simulink model "SimulatorSpencer"  (R2024a)
settings: Solver=VariableStepAuto  StartTime=0.0  StopTime=inf  MaxStep=1  RelTol=1e-5
model workspace (MAT data in the model file):
  A = 10
values from neighbouring files (symbols this model uses):
  CheckBox = modes(i)    [ACSModeSequence.m]    (also in Constants_gui.m = LampModes(i))
  I = [3000 0 0 ... (first row only)    [Constants_gui.m]    (also in constants.m; mbi.m = [15, .25, .20; set_up_HW7.m = I-Id; setupConstantRateSDA.m)
  invI = inv(I)    [Constants_gui.m]    (also in constants.m; mbi.m; set_up_HW7.m; setupConstantRateSDA.m)
  q_init = q_init/norm(q_init)    [Constants_gui.m]    (also in constants.m = [-0.5 -0.5 -0.5 0.5]; mbi.m = [0 0 0 1]'; set_up_HW7.m = [0 0 0 1]'; setupConstantRateSDA.m)
  wbn_init = pi/30*[0 0 0]'    [Constants_gui.m]    (also in constants.m = pi/180 * [0.1; 0.2; 0.15]; mbi.m = [0 0 0]'; set_up_HW7.m = pi/30*[0 0 .01]'; setupConstantRateSDA.m)
  wn = 0.01    [Constants_gui.m]    (also in constants.m = 0.05; setupConstantRateSDA.m = 0.05)
  zet = .7071    (= 0.7071)    [Constants_gui.m]    (also in constants.m; setupConstantRateSDA.m)
libraries: aerolibutil x9, sharedutil x8, sharedtransform x2, sldrtlib x1, dspinverses x1, vrlib x1
(part 3 of 4)

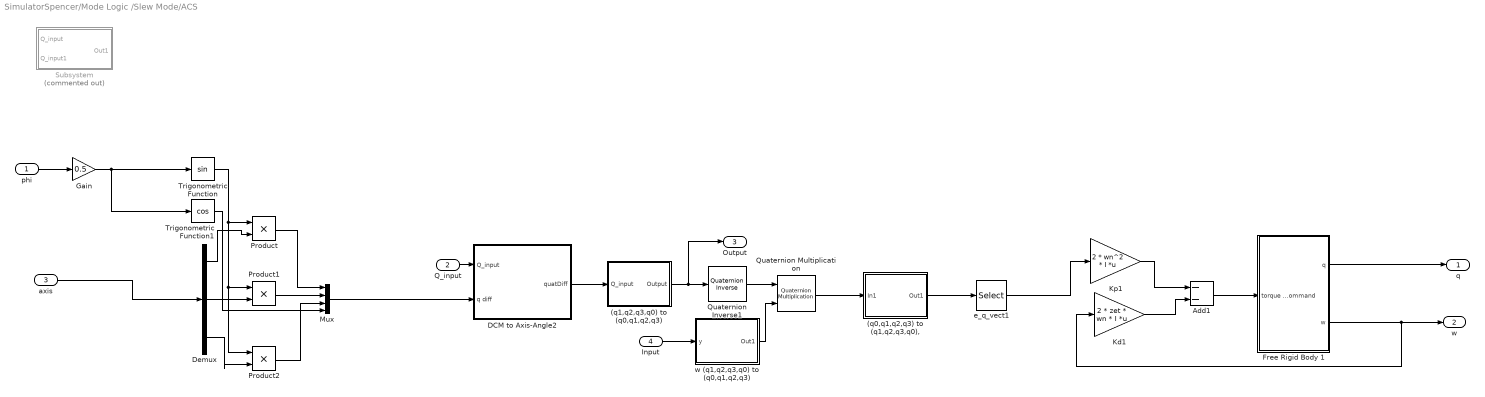
== system SimulatorSpencer/Mode Logic /Slew Mode/ACS ==
  phi : Inport
  Q_input : Inport  Port=2
  axis : Inport  Port=3
  Input : Inport  Port=4
  (q0,q1,q2,q3) to (q1,q2,q3,q0), : Subsystem
  "(q1,q2,q3,q0) to (q0,q1,q2,q3) " : Subsystem
  Add1 : Sum  Inputs=--
  DCM to Axis-Angle2 : Subsystem
  Demux : Demux  Outputs=3
  Free Rigid Body 1 : Subsystem
  Gain : Gain  Gain=0.5
  Kd1 : Gain  Gain=2 * zet * wn * I  Multiplication=Matrix(K*u)  SaturateOnIntegerOverflow=on  OutDataTypeStr=Inherit: Same as input  ParamDataTypeStr=Inherit: Same as input
  Kp1 : Gain  Gain=2 * wn^2 * I  Multiplication=Matrix(K*u)  SaturateOnIntegerOverflow=on  OutDataTypeStr=Inherit: Same as input  ParamDataTypeStr=Inherit: Same as input
  Mux : Mux
  Product : Product
  Product1 : Product
  Product2 : Product
  Quaternion Inverse1 : aerolibutil/Quaternion Inverse
  Quaternion Multiplication : aerolibutil/Quaternion Multiplication
  Subsystem : Subsystem  Commented=on
  Trigonometric Function : Trigonometry
  Trigonometric Function1 : Trigonometry  Operator=cos
  e_q_vect1 : Selector  InputPortWidth=4  IndexOptions=Index vector (dialog)  Indices=[1 2 3]  OutputSizes=1
  "w (q1,q2,q3,q0) to (q0,q1,q2,q3) " : Subsystem
      settings: PortSchema="{\"entries\":[{\"content\":{\"sides\":[{\"content\":{\"connectorIds\":[\"Out1\"]},\"type\":\"ConnectorPlacement.EquallySpacedRectSide\",\"uuid\":\"97b477ad-5663-4010-b344-d27b8ec095be\"},{\"content\":{\"connectorIds\":[\"In1\"],\"side\":\"RIGHT\"},\"type\":\"ConnectorPlacement.EquallySpacedRectSide\",\"uuid\":\"41fe4029-0263-4427-bdfc-3c26258b8a65\"},{\"content\":{\"side\":\"TOP\"},\"type\":\"ConnectorPlacement.EquallySpacedRectSide\",\"uuid\":\"9fb3a03d-539a-4245-bd7d-8174d3d0797f\"}]},\"type\":\"ConnectorPlacement.EquallySpacedConnector\",\"uuid\":\"44222554-f3ae-4bc6-b92c-7571a5ce84f7\"}],\"packageUris\":[\"http://schema.mathworks.com/mf0/Connector/R2020b\"],\"version\":\"1.0\"}"
  q : Outport
  w : Outport  Port=2
  Output : Outport  Port=3
  wires:
  Product1/1 -> Mux/2
  Product2/1 -> Mux/3
  Demux/1 -> Product/2
  Gain/1 -> Trigonometric Function1/1, Trigonometric Function/1
  Product/1 -> Mux/1
  phi/1 -> Gain/1
  Demux/2 -> Product1/2
  Demux/3 -> Product2/2
  Trigonometric Function1/1 -> Mux/4
  Trigonometric Function/1 -> Product2/1, Product1/1, Product/1
  axis/1 -> Demux/1
  Q_input/1 -> DCM to Axis-Angle2/1(Q_input)
  Mux/1 -> DCM to Axis-Angle2/2(q diff)
  Quaternion Multiplication/1 -> (q0,q1,q2,q3) to (q1,q2,q3,q0),/1(In1)
  "w (q1,q2,q3,q0) to (q0,q1,q2,q3) "/1(Out1) -> Quaternion Multiplication/2
  Quaternion Inverse1/1 -> Quaternion Multiplication/1
  Add1/1 -> Free Rigid Body 1/1(torque command)
  Kd1/1 -> Add1/2
  Free Rigid Body 1/2(w) -> w/1, Kd1/1
  "(q1,q2,q3,q0) to (q0,q1,q2,q3) "/1(Output) -> Output/1, Quaternion Inverse1/1
  e_q_vect1/1 -> Kp1/1
  DCM to Axis-Angle2/1(quatDiff) -> "(q1,q2,q3,q0) to (q0,q1,q2,q3) "/1(Q_input)
  (q0,q1,q2,q3) to (q1,q2,q3,q0),/1(Out1) -> e_q_vect1/1
  Kp1/1 -> Add1/1
  Free Rigid Body 1/1(q) -> q/1
  Input/1 -> "w (q1,q2,q3,q0) to (q0,q1,q2,q3) "/1(y)

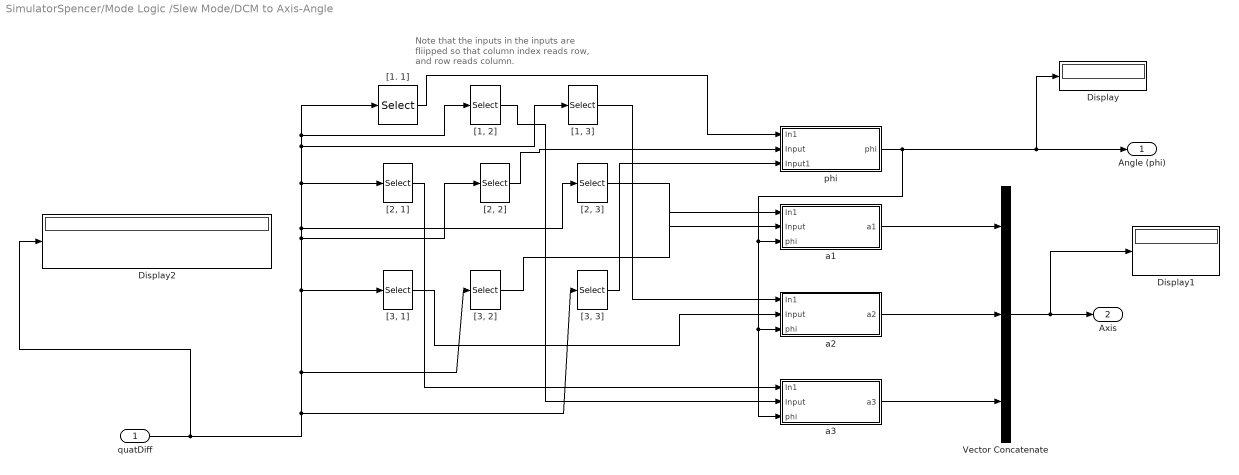
== system SimulatorSpencer/Mode Logic /Slew Mode/DCM to Axis-Angle ==
  note: Note that the inputs in the inputs are fliipped so that column index reads row, and row reads column.
  quatDiff : Inport
  Display : Display
  Display1 : Display
  Display2 : Display
  Vector Concatenate : Concatenate  NumInputs=3
  "[1, 2]" : Selector  NumberOfDimensions=2  InputPortWidth=3  IndexOptions=Index vector (dialog),Index vector (dialog)  Indices=2,1  OutputSizes=1,1
  "[1, 3]" : Selector  NumberOfDimensions=2  InputPortWidth=3  IndexOptions=Index vector (dialog),Index vector (dialog)  Indices=3,1  OutputSizes=1,1
  "[1. 1]" : Selector  NumberOfDimensions=2  InputPortWidth=3  IndexOptions=Index vector (dialog),Index vector (dialog)  Indices=1,1  OutputSizes=1,1
  "[2, 1]" : Selector  NumberOfDimensions=2  InputPortWidth=3  IndexOptions=Index vector (dialog),Index vector (dialog)  Indices=1,2  OutputSizes=1,1
  "[2, 2]" : Selector  NumberOfDimensions=2  InputPortWidth=3  IndexOptions=Index vector (dialog),Index vector (dialog)  Indices=2,2  OutputSizes=1,1
  "[2, 3]" : Selector  NumberOfDimensions=2  InputPortWidth=3  IndexOptions=Index vector (dialog),Index vector (dialog)  Indices=3,2  OutputSizes=1,1
  "[3, 1]" : Selector  NumberOfDimensions=2  InputPortWidth=3  IndexOptions=Index vector (dialog),Index vector (dialog)  Indices=1,3  OutputSizes=1,1
  "[3, 2]" : Selector  NumberOfDimensions=2  InputPortWidth=3  IndexOptions=Index vector (dialog),Index vector (dialog)  Indices=2,3  OutputSizes=1,1
  "[3, 3]" : Selector  NumberOfDimensions=2  InputPortWidth=3  IndexOptions=Index vector (dialog),Index vector (dialog)  Indices=3,3  OutputSizes=1,1
  a1 : Subsystem
  a2 : Subsystem
  a3 : Subsystem
  phi : Subsystem
  Angle (phi) : Outport
  Axis : Outport  Port=2
  wires:
  Vector Concatenate/1 -> Display1/1, Axis/1
  "[3, 3]"/1 -> phi/3(Input1)
  "[2, 3]"/1 -> a1/2(Input)
  "[1, 3]"/1 -> a2/1(In1)
  a2/1(a2) -> Vector Concatenate/2
  "[2, 2]"/1 -> phi/2(Input)
  "[1, 2]"/1 -> a3/2(Input)
  "[1. 1]"/1 -> phi/1(In1)
  "[2, 1]"/1 -> a3/1(In1)
  "[3, 1]"/1 -> a2/2(Input)
  "[3, 2]"/1 -> a1/1(In1)
  quatDiff/1 -> Display2/1, "[3, 2]"/1, "[3, 1]"/1, "[2, 1]"/1, "[1, 3]"/1, "[1, 2]"/1, "[1. 1]"/1, "[2, 3]"/1, "[2, 2]"/1, "[3, 3]"/1
  phi/1(phi) -> Angle (phi)/1, Display/1, a3/3(phi), a2/3(phi), a1/3(phi)
  a3/1(a3) -> Vector Concatenate/3
  a1/1(a1) -> Vector Concatenate/1

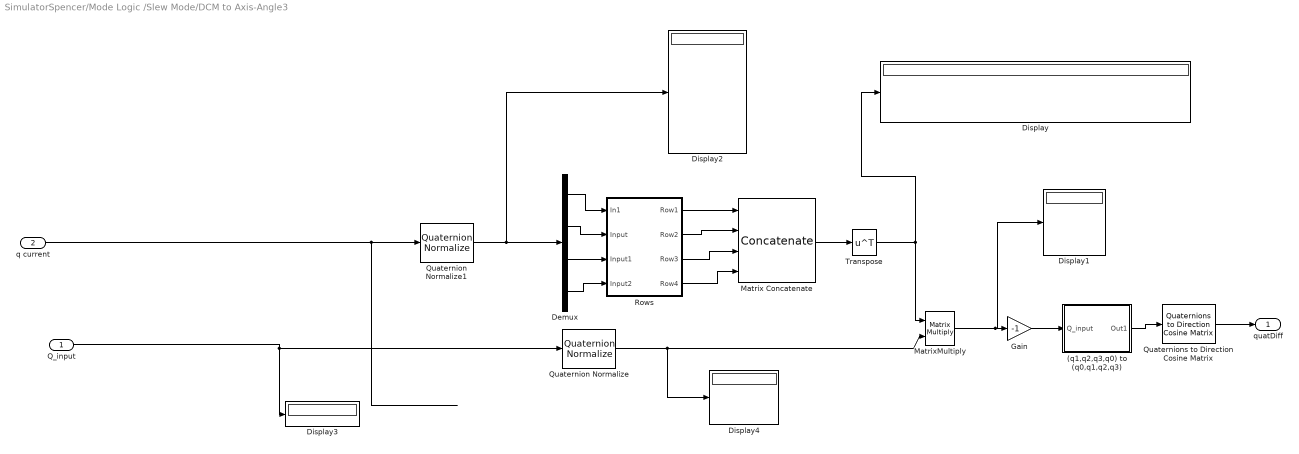
== system SimulatorSpencer/Mode Logic /Slew Mode/DCM to Axis-Angle3 ==
  Q_input : Inport
  q current : Inport  Port=2
  "(q1,q2,q3,q0) to (q0,q1,q2,q3) " : Subsystem
  Demux : Demux
  Display{,1..4} (5 alike) : Display
  Gain : Gain  Gain=-1
  Matrix Concatenate : Concatenate  NumInputs=4  Mode=Multidimensional array  ConcatenateDimension=2
  MatrixMultiply : Product  Multiplication=Matrix(*)
  Quaternion Normalize : sharedutil/Quaternion Normalize  aMode=aMode
  Quaternion Normalize1 : sharedutil/Quaternion Normalize  aMode=aMode
  Quaternions to Direction Cosine Matrix : sharedtransform/Quaternions to  Direction Cosine Matrix  aMode=aMode
      settings: LibrarySourceBlock=|
      | aerolibtransform2/Quaternions to
      | Direction Cosine Matrix
  Rows : Subsystem
  Transpose : Math  Operator=transpose
  quatDiff : Outport
  wires:
  Rows/1(Row1) -> Matrix Concatenate/1
  Rows/2(Row2) -> Matrix Concatenate/2
  Rows/3(Row3) -> Matrix Concatenate/3
  Rows/4(Row4) -> Matrix Concatenate/4
  Demux/1 -> Rows/1(In1)
  Demux/2 -> Rows/2(Input)
  Demux/3 -> Rows/3(Input1)
  Demux/4 -> Rows/4(Input2)
  Matrix Concatenate/1 -> Transpose/1
  Transpose/1 -> MatrixMultiply/1, Display/1
  MatrixMultiply/1 -> Gain/1, Display1/1
  Q_input/1 -> Quaternion Normalize/1, Display3/1
  q current/1 -> Quaternion Normalize1/1
  Quaternions to Direction Cosine Matrix/1 -> quatDiff/1
  Gain/1 -> "(q1,q2,q3,q0) to (q0,q1,q2,q3) "/1(Q_input)
  "(q1,q2,q3,q0) to (q0,q1,q2,q3) "/1(Out1) -> Quaternions to Direction Cosine Matrix/1
  Quaternion Normalize/1 -> Display4/1, MatrixMultiply/2
  Quaternion Normalize1/1 -> Display2/1, Demux/1

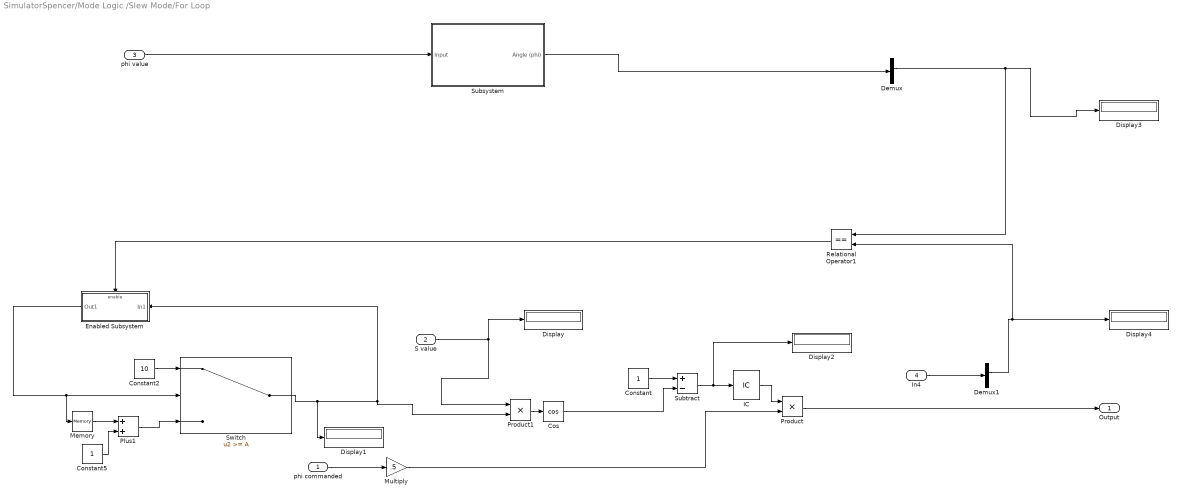
== system SimulatorSpencer/Mode Logic /Slew Mode/For Loop ==
  phi commanded : Inport
  S value : Inport  Port=2
  phi value : Inport  Port=3
  In4 : Inport  Port=4
  Constant : Constant
  Constant2 : Constant  Value=10
  Constant5 : Constant
  Cos : Trigonometry  Operator=cos
  Demux : Demux
  Demux1 : Demux
  Display{,1..4} (5 alike) : Display
      Display3 settings: Decimation=10000
      Display4 settings: Decimation=100000
  Enabled Subsystem : Subsystem  TreatAsAtomicUnit=on
  IC : InitialCondition  Value=0
  Memory : Memory  InitialCondition=-1
  Multiply : Gain  Gain=.5
  Plus1 : Sum
  Product : Product
  Product1 : Product
  Relational Operator1 : RelationalOperator  Operator===  OutDataTypeStr=boolean  RndMeth=Simplest  InputSameDT=off
  Subsystem : Subsystem
  Subtract : Sum  Inputs=+-
  Switch : Switch  Threshold=A  ZeroCross=off  SaturateOnIntegerOverflow=off  InputSameDT=off
  Output : Outport
  wires:
  Constant2/1 -> Switch/1
  Plus1/1 -> Switch/3
  Constant5/1 -> Plus1/2
  Product1/1 -> Cos/1
  Constant/1 -> Subtract/1
  Cos/1 -> Subtract/2
  Subtract/1 -> IC/1, Display2/1
  phi commanded/1 -> Multiply/1
  Multiply/1 -> Product/2
  Product/1 -> Output/1
  S value/1 -> Product1/1, Display/1
  Switch/1 -> Display1/1, Enabled Subsystem/1(In1), Product1/2
  IC/1 -> Product/1
  Memory/1 -> Plus1/1
  In4/1 -> Demux1/1
  Enabled Subsystem/1(Out1) -> Switch/2, Memory/1
  phi value/1 -> Subsystem/1(Input)
  Demux/2 -> Relational Operator1/1, Display3/1
  Demux1/2 -> Relational Operator1/2, Display4/1
  Relational Operator1/1 -> Enabled Subsystem/Enable
  Subsystem/1(Angle (phi)) -> Demux/1

== system SimulatorSpencer/Mode Logic /Slew Mode/Subsystem ==
  Axis : Inport
  Divide : Product  Inputs=*/
  Integrator : Integrator  Commented=on
  Quaternion Integration : Subsystem  Commented=on
  S : Subsystem
  T : Constant  Value=10
  acceleration : Subsystem  Commented=on
  invI : Gain  Commented=on  Gain=invI  Multiplication=Matrix(K*u)
  S value : Outport
  wires:
  S/1(Out1) -> S value/1
  Integrator/1 -> Quaternion Integration/1(w_Body)
  Quaternion Integration/1(q_I_Body) -> ?
  ? -> acceleration/3(tcurrent)
  ? -> S/1(Input), acceleration/2(tnot)
  Axis/1 -> acceleration/5(Axis)
  invI/1 -> Integrator/1
  acceleration/1(Spacecraft torque) -> invI/1
  T/1 -> Divide/2
  Divide/1 -> ?

== system SimulatorSpencer/Mode Selection/Commanded values/Commanded Quaternion ==
  Constant : Constant  Value=99
  Constant1 : Constant  Value=4
  Constant2 : Constant  Value=10
  Constant3 : Constant  Value=4
  Vector Concatenate : Concatenate  NumInputs=4
  Out1 : Outport
  wires:
  Constant2/1 -> Vector Concatenate/1
  Constant3/1 -> Vector Concatenate/4
  Vector Concatenate/1 -> Out1/1
  Constant1/1 -> Vector Concatenate/3
  Constant/1 -> Vector Concatenate/2

== system SimulatorSpencer/Mode Selection/Commanded values/Commanded Quaternion1 ==
  note: TURN ON INITAL CONDITIONS
  Constant : Constant  Value=0
  Constant1 : Constant  Value=0
  Constant2 : Constant  Value=0
  Constant3 : Constant
  Normalize Vector : vrlib/Utilities/Normalize Vector  maxzero=0
  Slider Switch1 : CustomTuningWebBlock  LabelPosition=Hide  ShowInitialText=on  Configuration="{\"components\":[{\"name\":\"CustomSwitchStateComponent\",\"settings\":{\"position\":[0,0,1,1],\"states\":[{\"HitRegion\":{\"position\":[0,0,0.5,1]},\"Image\":{\"position\":[0,0,1,1],\"size\":[1,1],\"src\":\"data:image\\/svg+xml;base64,PD94bWwgdmVyc2lvbj0iMS4wIiBlbmNvZGluZz0idXRmLTgiPz4NCjwhLS0gR2VuZXJhdG9yOiBBZG9iZSBJbGx1c3RyYXRvciAyNS4yLjEsIFNWRyBFeHBvcnQgUGx1Zy1JbiAuIFNWRyBWZXJzaW9uOiA2LjAwIEJ1aWxkIDApICAtLT4NCjxzdmcgdmVyc2lvbj0iMS4xIiB4bWxucz0iaHR0cDovL3d3dy53My5vcmcvMjAwMC9zdmciIHhtbG5zOnhsaW5rPSJodHRwOi8vd3d3LnczLm9yZy8xOTk5L3hsaW5rIiB4PSIwcHgiIHk9IjBweCINCgkgdmlld0JveD0iMCAwIDc2IDI5IiBzdHlsZT0iZW5hYmxlLWJhY2tncm91bmQ6bmV3 ...(+5404 chars)\",\"srcOrientation\":\"Right\"},\"Label\":{\"color\":[0.9882352941176471,0.9882352941176471,0.7725490196078432],\"icon\":{\"size\":[0,0],\"src\":[],\"srcOrientation\":\"Right\"},\"iconPlacement\":\"left\",\"opacity\":1,\"position\":[0.5,0.14],\"show\":true,\"text\":{\"content\":\"Off\",\"font\":\"Helvetica\",\"fontSize\":7}},\"Value\":0},{\"HitRegion\":{\"position\":[0,0.5,0.5,1]},\"Image\":{\"position\":[0,0,1,1],\"size\":[1,1],\"src\":\"data:image\\/svg+xml;base64,PD94bWwgdmVyc2lvbj0iMS4wIiBlbmNvZGluZz0idXRmLTgiPz4NCjwhLS0gR2VuZXJhdG9yOiBBZG9iZSBJbGx1c3RyYXRvciAyNS4yLjEsIFNWRyBFeHBvcnQgUGx1Zy1JbiAuIFNWRyBWZXJzaW9uOiA2LjAwIEJ1aWxkIDApICAtLT4NCjxzdmcgdmVyc2lvbj0iMS4xIiB4bWxucz0iaHR0cDovL3d3dy53My5vcmcvMjAwMC9zdmciIHhtbG5zOnhsaW5rPSJodHRwOi8vd3d3LnczLm9yZy8xOTk5L3hsaW5rIiB4PSIwcHgiIHk9IjBweCINCgkgdmlld0JveD0iMCAwIDc2IDI5IiBzdHlsZT0iZW5hYmxlLWJhY2tncm91bmQ6bmV3 ...(+5404 chars)\",\"srcOrientation\":\"Right\"},\"Label\":{\"color\":[0.9882352941176471,0.9882352941176471,0.7725490196078432],\"icon\":{\"size\":[0,0],\"src\":[],\"srcOrientation\":\"Right\"},\"iconPlacement\":\"left\",\"opacity\":1,\"position\":[0.5,0.86],\"show\":true,\"text\":{\"content\":\"On\",\"font\":\"Helvetica\",\"fontSize\":7}},\"Value\":1}]}},{\"name\":\"BackgroundImageComponent\",\"settings\":{\"image\":{\"size\":[140,55],\"src\":\"default\",\"srcOrientation\":\"Right\"},\"position\":[0,0,1,1],\"scaleMode\":\"0\"}},{\"name\":\"ForegroundImageComponent\",\"settings\":{\"image\":{\"size\":[0,0],\"src\":\"default\",\"srcOrientation\":[]},\"isForeground\":1,\"position\":[0,0,1,1],\"scaleMode\":\"0\"}}],\"settings\":{\"BindingType\":\"param\",\"backgroundColor\":[0,0,255,\"1\"],\"backgroundOffset\":0.14,\"fixedAspectRatio\":\"on\",\"foregroundColor\":[234,234,234],\"showBackgroundColor\":false,\"variant\":\"slider\",\"version\":\"R2023a\"},\"type\":\"Switch\"}"
  Vector Concatenate : Concatenate  NumInputs=4
  QUaternion : Outport
  wires:
  Constant2/1 -> Vector Concatenate/1
  Constant3/1 -> Vector Concatenate/4
  Vector Concatenate/1 -> Normalize Vector/1
  Constant1/1 -> Vector Concatenate/3
  Constant/1 -> Vector Concatenate/2
  Normalize Vector/1 -> QUaternion/1

== system SimulatorSpencer/Mode Selection/Commanded values/Commanded Velocity ==
  Constant : Constant
  Constant1 : Constant
  Constant2 : Constant
  Vector Concatenate : Concatenate  NumInputs=3
  Out1 : Outport
  wires:
  Constant/1 -> Vector Concatenate/2
  Constant1/1 -> Vector Concatenate/3
  Vector Concatenate/1 -> Out1/1
  Constant2/1 -> Vector Concatenate/1

== system SimulatorSpencer/Mode Logic /ACS/Free Rigid Body 1/Cross ==
  A : Inport
  B : Inport  Port=2
  Mux4 : Mux  Inputs=3
  Product{,1..5} (6 alike) : Product  InputSameDT=on  SaturateOnIntegerOverflow=on  OutDataTypeStr=Inherit: Same as first input
  Sum : Sum  Inputs=+-  InputSameDT=on  SaturateOnIntegerOverflow=on  OutDataTypeStr=Inherit: Same as first input
  Sum1 : Sum  Inputs=+-  InputSameDT=on  SaturateOnIntegerOverflow=on  OutDataTypeStr=Inherit: Same as first input
  Sum2 : Sum  Inputs=+-  InputSameDT=on  SaturateOnIntegerOverflow=on  OutDataTypeStr=Inherit: Same as first input
  demux2 : Demux  Outputs=3
      settings: DisplayOption=none
  demux3 : Demux  Outputs=3
      settings: DisplayOption=none
  AxB : Outport  InitialOutput=0
  wires:
  A/1 -> demux2/1
  B/1 -> demux3/1
  demux2/3 -> Product1/1, Product2/1
  demux3/3 -> Product/2, Product3/2
  demux2/1 -> Product3/1, Product4/1
  demux3/2 -> Product1/2, Product4/2
  demux2/2 -> Product/1, Product5/1
  demux3/1 -> Product2/2, Product5/2
  Product/1 -> Sum/1
  Product1/1 -> Sum/2
  Product2/1 -> Sum1/1
  Product3/1 -> Sum1/2
  Product4/1 -> Sum2/1
  Product5/1 -> Sum2/2
  Sum/1 -> Mux4/1
  Sum1/1 -> Mux4/2
  Sum2/1 -> Mux4/3
  Mux4/1 -> AxB/1

== system SimulatorSpencer/Mode Logic /ACS/Free Rigid Body 1/Quaternion Integration ==
  w_Body : Inport
  Integrator1 : Integrator  InitialCondition=q_init
  q_normalize : Subsystem
  qderiv : Subsystem
  q_I_Body : Outport
  wires:
  w_Body/1 -> qderiv/1(w)
  q_normalize/1(q_out) -> qderiv/2(q), q_I_Body/1
  Integrator1/1 -> q_normalize/1(q_in)
  qderiv/1(qd) -> Integrator1/1

== system SimulatorSpencer/Mode Logic /ACS/Free Rigid Body 1/Subsystem ==
  q1 q2 q3 q4 : Inport
  Demux : Demux
      settings: DisplayOption=none
  Gain1 : Gain  Gain=2  SaturateOnIntegerOverflow=on  OutDataTypeStr=Inherit: Same as input  ParamDataTypeStr=Inherit: Same as input
  Gain2 : Gain  Gain=2  SaturateOnIntegerOverflow=on  OutDataTypeStr=Inherit: Same as input  ParamDataTypeStr=Inherit: Same as input
  Matrix Gain : Gain  Gain=eye(3,3)  SaturateOnIntegerOverflow=on  OutDataTypeStr=Inherit: Same as input  ParamDataTypeStr=Inherit: Same as input
  Mux : Mux  Inputs=3
  Product : Product  InputSameDT=on  SaturateOnIntegerOverflow=on  OutDataTypeStr=Inherit: Same as first input
  Product1 : Product  InputSameDT=on  SaturateOnIntegerOverflow=on  OutDataTypeStr=Inherit: Same as first input
  Subsystem : Subsystem
      mask Display: disp('3x3 cross matrix')
  Sum1 : Sum  Inputs=|+-  InputSameDT=on  SaturateOnIntegerOverflow=on  OutDataTypeStr=Inherit: Same as first input
  Sum8 : Sum  Inputs=|+-+  InputSameDT=on  SaturateOnIntegerOverflow=on  OutDataTypeStr=Inherit: Same as first input
  T1 : Math  Operator=transpose  SignedPower=on
  T2 : Math  Operator=transpose  SignedPower=on
  qTq : Product  Multiplication=Matrix(*)  InputSameDT=on  SaturateOnIntegerOverflow=on  OutDataTypeStr=Inherit: Same as first input
  qqT : Product  Multiplication=Matrix(*)  InputSameDT=on  SaturateOnIntegerOverflow=on  OutDataTypeStr=Inherit: Same as first input
  DCM : Outport  InitialOutput=0
  wires:
  T1/1 -> qqT/2
  Sum8/1 -> DCM/1
  Product/1 -> Gain1/1
  Demux/3 -> Mux/3
  Demux/2 -> Mux/2
  qqT/1 -> Gain2/1
  Gain1/1 -> Sum8/2
  q1 q2 q3 q4/1 -> Demux/1
  Demux/1 -> Mux/1
  Matrix Gain/1 -> Sum8/3
  Product1/1 -> Sum1/1
  qTq/1 -> Sum1/2
  T2/1 -> qTq/1
  Subsystem/1(Out1) -> Product/1
  Mux/1 -> qTq/2, T2/1, qqT/1, T1/1, Subsystem/1(In1)
  Demux/4 -> Product1/2, Product1/1, Product/2
  Sum1/1 -> Matrix Gain/1
  Gain2/1 -> Sum8/1

== system SimulatorSpencer/Mode Logic /Constant Rate Mode/Free Rigid Body /Cross ==
  A : Inport
  B : Inport  Port=2
  Mux4 : Mux  Inputs=3
  Product{,1..5} (6 alike) : Product  InputSameDT=on  SaturateOnIntegerOverflow=on  OutDataTypeStr=Inherit: Same as first input
  Sum : Sum  Inputs=+-  InputSameDT=on  SaturateOnIntegerOverflow=on  OutDataTypeStr=Inherit: Same as first input
  Sum1 : Sum  Inputs=+-  InputSameDT=on  SaturateOnIntegerOverflow=on  OutDataTypeStr=Inherit: Same as first input
  Sum2 : Sum  Inputs=+-  InputSameDT=on  SaturateOnIntegerOverflow=on  OutDataTypeStr=Inherit: Same as first input
  demux2 : Demux  Outputs=3
      settings: DisplayOption=none
  demux3 : Demux  Outputs=3
      settings: DisplayOption=none
  AxB : Outport  InitialOutput=0
  wires:
  A/1 -> demux2/1
  B/1 -> demux3/1
  demux2/3 -> Product1/1, Product2/1
  demux3/3 -> Product/2, Product3/2
  demux2/1 -> Product3/1, Product4/1
  demux3/2 -> Product1/2, Product4/2
  demux2/2 -> Product/1, Product5/1
  demux3/1 -> Product2/2, Product5/2
  Product/1 -> Sum/1
  Product1/1 -> Sum/2
  Product2/1 -> Sum1/1
  Product3/1 -> Sum1/2
  Product4/1 -> Sum2/1
  Product5/1 -> Sum2/2
  Sum/1 -> Mux4/1
  Sum1/1 -> Mux4/2
  Sum2/1 -> Mux4/3
  Mux4/1 -> AxB/1

== system SimulatorSpencer/Mode Logic /Constant Rate Mode/Free Rigid Body /Quaternion Integration ==
  w_Body : Inport
  Integrator1 : Integrator  InitialCondition=q_init
  q_normalize : Subsystem
  qderiv : Subsystem
  q_I_Body : Outport
  wires:
  w_Body/1 -> qderiv/1(w)
  q_normalize/1(q_out) -> qderiv/2(q), q_I_Body/1
  Integrator1/1 -> q_normalize/1(q_in)
  qderiv/1(qd) -> Integrator1/1

== system SimulatorSpencer/Mode Logic /Constant Rate Mode/Free Rigid Body /Subsystem ==
  q1 q2 q3 q4 : Inport
  Demux : Demux
      settings: DisplayOption=none
  Gain1 : Gain  Gain=2  SaturateOnIntegerOverflow=on  OutDataTypeStr=Inherit: Same as input  ParamDataTypeStr=Inherit: Same as input
  Gain2 : Gain  Gain=2  SaturateOnIntegerOverflow=on  OutDataTypeStr=Inherit: Same as input  ParamDataTypeStr=Inherit: Same as input
  Matrix Gain : Gain  Gain=eye(3,3)  SaturateOnIntegerOverflow=on  OutDataTypeStr=Inherit: Same as input  ParamDataTypeStr=Inherit: Same as input
  Mux : Mux  Inputs=3
  Product : Product  InputSameDT=on  SaturateOnIntegerOverflow=on  OutDataTypeStr=Inherit: Same as first input
  Product1 : Product  InputSameDT=on  SaturateOnIntegerOverflow=on  OutDataTypeStr=Inherit: Same as first input
  Subsystem : Subsystem
      mask Display: disp('3x3 cross matrix')
  Sum1 : Sum  Inputs=|+-  InputSameDT=on  SaturateOnIntegerOverflow=on  OutDataTypeStr=Inherit: Same as first input
  Sum8 : Sum  Inputs=|+-+  InputSameDT=on  SaturateOnIntegerOverflow=on  OutDataTypeStr=Inherit: Same as first input
  T1 : Math  Operator=transpose  SignedPower=on
  T2 : Math  Operator=transpose  SignedPower=on
  qTq : Product  Multiplication=Matrix(*)  InputSameDT=on  SaturateOnIntegerOverflow=on  OutDataTypeStr=Inherit: Same as first input
  qqT : Product  Multiplication=Matrix(*)  InputSameDT=on  SaturateOnIntegerOverflow=on  OutDataTypeStr=Inherit: Same as first input
  DCM : Outport  InitialOutput=0
  wires:
  T1/1 -> qqT/2
  Sum8/1 -> DCM/1
  Product/1 -> Gain1/1
  Demux/3 -> Mux/3
  Demux/2 -> Mux/2
  qqT/1 -> Gain2/1
  Gain1/1 -> Sum8/2
  q1 q2 q3 q4/1 -> Demux/1
  Demux/1 -> Mux/1
  Matrix Gain/1 -> Sum8/3
  Product1/1 -> Sum1/1
  qTq/1 -> Sum1/2
  T2/1 -> qTq/1
  Subsystem/1(Out1) -> Product/1
  Mux/1 -> qTq/2, T2/1, qqT/1, T1/1, Subsystem/1(In1)
  Demux/4 -> Product1/2, Product1/1, Product/2
  Sum1/1 -> Matrix Gain/1
  Gain2/1 -> Sum8/1

== system SimulatorSpencer/Mode Logic /Momentum Dump/Free Rigid Body 1/Cross ==
  A : Inport
  B : Inport  Port=2
  Mux4 : Mux  Inputs=3
  Product{,1..5} (6 alike) : Product  InputSameDT=on  SaturateOnIntegerOverflow=on  OutDataTypeStr=Inherit: Same as first input
  Sum : Sum  Inputs=+-  InputSameDT=on  SaturateOnIntegerOverflow=on  OutDataTypeStr=Inherit: Same as first input
  Sum1 : Sum  Inputs=+-  InputSameDT=on  SaturateOnIntegerOverflow=on  OutDataTypeStr=Inherit: Same as first input
  Sum2 : Sum  Inputs=+-  InputSameDT=on  SaturateOnIntegerOverflow=on  OutDataTypeStr=Inherit: Same as first input
  demux2 : Demux  Outputs=3
      settings: DisplayOption=none
  demux3 : Demux  Outputs=3
      settings: DisplayOption=none
  AxB : Outport  InitialOutput=0
  wires:
  A/1 -> demux2/1
  B/1 -> demux3/1
  demux2/3 -> Product1/1, Product2/1
  demux3/3 -> Product/2, Product3/2
  demux2/1 -> Product3/1, Product4/1
  demux3/2 -> Product1/2, Product4/2
  demux2/2 -> Product/1, Product5/1
  demux3/1 -> Product2/2, Product5/2
  Product/1 -> Sum/1
  Product1/1 -> Sum/2
  Product2/1 -> Sum1/1
  Product3/1 -> Sum1/2
  Product4/1 -> Sum2/1
  Product5/1 -> Sum2/2
  Sum/1 -> Mux4/1
  Sum1/1 -> Mux4/2
  Sum2/1 -> Mux4/3
  Mux4/1 -> AxB/1

== system SimulatorSpencer/Mode Logic /Momentum Dump/Free Rigid Body 1/Quaternion Integration ==
  w_Body : Inport
  Integrator1 : Integrator  InitialCondition=q_init
  q_normalize : Subsystem
  qderiv : Subsystem
  q_I_Body : Outport
  wires:
  w_Body/1 -> qderiv/1(w)
  q_normalize/1(q_out) -> qderiv/2(q), q_I_Body/1
  Integrator1/1 -> q_normalize/1(q_in)
  qderiv/1(qd) -> Integrator1/1

== system SimulatorSpencer/Mode Logic /Momentum Dump/Free Rigid Body 1/Subsystem ==
  q1 q2 q3 q4 : Inport
  Demux : Demux
      settings: DisplayOption=none
  Gain1 : Gain  Gain=2  SaturateOnIntegerOverflow=on  OutDataTypeStr=Inherit: Same as input  ParamDataTypeStr=Inherit: Same as input
  Gain2 : Gain  Gain=2  SaturateOnIntegerOverflow=on  OutDataTypeStr=Inherit: Same as input  ParamDataTypeStr=Inherit: Same as input
  Matrix Gain : Gain  Gain=eye(3,3)  SaturateOnIntegerOverflow=on  OutDataTypeStr=Inherit: Same as input  ParamDataTypeStr=Inherit: Same as input
  Mux : Mux  Inputs=3
  Product : Product  InputSameDT=on  SaturateOnIntegerOverflow=on  OutDataTypeStr=Inherit: Same as first input
  Product1 : Product  InputSameDT=on  SaturateOnIntegerOverflow=on  OutDataTypeStr=Inherit: Same as first input
  Subsystem : Subsystem
      mask Display: disp('3x3 cross matrix')
  Sum1 : Sum  Inputs=|+-  InputSameDT=on  SaturateOnIntegerOverflow=on  OutDataTypeStr=Inherit: Same as first input
  Sum8 : Sum  Inputs=|+-+  InputSameDT=on  SaturateOnIntegerOverflow=on  OutDataTypeStr=Inherit: Same as first input
  T1 : Math  Operator=transpose  SignedPower=on
  T2 : Math  Operator=transpose  SignedPower=on
  qTq : Product  Multiplication=Matrix(*)  InputSameDT=on  SaturateOnIntegerOverflow=on  OutDataTypeStr=Inherit: Same as first input
  qqT : Product  Multiplication=Matrix(*)  InputSameDT=on  SaturateOnIntegerOverflow=on  OutDataTypeStr=Inherit: Same as first input
  DCM : Outport  InitialOutput=0
  wires:
  T1/1 -> qqT/2
  Sum8/1 -> DCM/1
  Product/1 -> Gain1/1
  Demux/3 -> Mux/3
  Demux/2 -> Mux/2
  qqT/1 -> Gain2/1
  Gain1/1 -> Sum8/2
  q1 q2 q3 q4/1 -> Demux/1
  Demux/1 -> Mux/1
  Matrix Gain/1 -> Sum8/3
  Product1/1 -> Sum1/1
  qTq/1 -> Sum1/2
  T2/1 -> qTq/1
  Subsystem/1(Out1) -> Product/1
  Mux/1 -> qTq/2, T2/1, qqT/1, T1/1, Subsystem/1(In1)
  Demux/4 -> Product1/2, Product1/1, Product/2
  Sum1/1 -> Matrix Gain/1
  Gain2/1 -> Sum8/1

== system SimulatorSpencer/Mode Logic /Slew Mode/ACS/(q0,q1,q2,q3) to (q1,q2,q3,q0), ==
  In1 : Inport
  Display : Display
  Display1 : Display
  Vector Concatenate : Concatenate
  e_q_vect1 : Selector  InputPortWidth=4  IndexOptions=Index vector (dialog)  Indices=[2 3 4]  OutputSizes=1
  e_q_vect2 : Selector  InputPortWidth=4  IndexOptions=Index vector (dialog)  Indices=[1]  OutputSizes=1
  Out1 : Outport
  wires:
  Vector Concatenate/1 -> Display1/1, Out1/1
  In1/1 -> Display/1, e_q_vect2/1, e_q_vect1/1
  e_q_vect1/1 -> Vector Concatenate/1
  e_q_vect2/1 -> Vector Concatenate/2

== system SimulatorSpencer/Mode Logic /Slew Mode/ACS/(q1,q2,q3,q0) to (q0,q1,q2,q3)  ==
  Q_input : Inport
  Quaternion Normalize : sharedutil/Quaternion Normalize  aMode=aMode
  Vector Concatenate : Concatenate
  e_q_vect1 : Selector  InputPortWidth=4  IndexOptions=Index vector (dialog)  Indices=[1 2 3]  OutputSizes=1
  e_q_vect2 : Selector  InputPortWidth=4  IndexOptions=Index vector (dialog)  Indices=[4]  OutputSizes=1
  Output : Outport
  wires:
  Q_input/1 -> e_q_vect2/1, e_q_vect1/1
  e_q_vect2/1 -> Vector Concatenate/1
  e_q_vect1/1 -> Vector Concatenate/2
  Vector Concatenate/1 -> Quaternion Normalize/1
  Quaternion Normalize/1 -> Output/1

== system SimulatorSpencer/Mode Logic /Slew Mode/ACS/DCM to Axis-Angle2 ==
  Q_input : Inport
  q diff : Inport  Port=2
  Demux : Demux
  Display : Display
  Display1 : Display
  Display3 : Display
  Matrix Concatenate : Concatenate  NumInputs=4  Mode=Multidimensional array  ConcatenateDimension=2
  MatrixMultiply : Product  Multiplication=Matrix(*)
  Rows : Subsystem
  Transpose : Math  Operator=transpose
  quatDiff : Outport
  wires:
  Rows/1(Row1) -> Matrix Concatenate/1
  Rows/2(Row2) -> Matrix Concatenate/2
  Rows/3(Row3) -> Matrix Concatenate/3
  Rows/4(Row4) -> Matrix Concatenate/4
  Demux/1 -> Rows/1(In1)
  Demux/2 -> Rows/2(Input)
  Demux/3 -> Rows/3(Input1)
  Demux/4 -> Rows/4(Input2)
  Matrix Concatenate/1 -> Transpose/1
  Transpose/1 -> MatrixMultiply/1, Display/1
  Q_input/1 -> Demux/1
  MatrixMultiply/1 -> quatDiff/1, Display1/1
  q diff/1 -> Display3/1, MatrixMultiply/2

== system SimulatorSpencer/Mode Logic /Slew Mode/ACS/Free Rigid Body 1 ==
  torque command : Inport
  Cross : Subsystem
  DCM : ToWorkspace  Commented=on  VariableName=DCM  SaveFormat=Structure With Time  SampleTime=-1
  Inertia : Gain  Gain=I  Multiplication=Matrix(K*u)  SaturateOnIntegerOverflow=on  OutDataTypeStr=Inherit: Same as input  ParamDataTypeStr=Inherit: Same as input
  Isc inverse : Gain  Gain=invI  Multiplication=Matrix(K*u)  SaturateOnIntegerOverflow=on  OutDataTypeStr=Inherit: Same as input  ParamDataTypeStr=Inherit: Same as input
  Quaternion Integration : Subsystem
  Subsystem : Subsystem  Commented=on
  Sum : Sum  Inputs=|+-  InputSameDT=on  SaturateOnIntegerOverflow=on  OutDataTypeStr=Inherit: Same as first input
  "wdot -> w" : Integrator  InitialCondition=wbn_init
  q : Outport
  w : Outport  Port=2
  wires:
  "wdot -> w"/1 -> w/1, Quaternion Integration/1(w_Body), Inertia/1, Cross/1(A)
  Sum/1 -> Isc inverse/1
  torque command/1 -> Sum/1
  Cross/1(AxB) -> Sum/2
  Inertia/1 -> Cross/2(B)
  Quaternion Integration/1(q_I_Body) -> Subsystem/1(q1 q2 q3 q4), q/1
  Subsystem/1(DCM) -> DCM/1
  Isc inverse/1 -> "wdot -> w"/1

== system SimulatorSpencer/Mode Logic /Slew Mode/ACS/Subsystem ==
  Q_input : Inport
  Q_input1 : Inport  Port=2
  (q0,q1,q2,q3) to (q1,q2,q3,q0), : Subsystem
  "(q1,q2,q3,q0) to (q0,q1,q2,q3) " : Subsystem
  (q1,q2,q3,q0) to (q0,q1,q2,q3) 1 : Subsystem
  Quaternion Multiplication : aerolibutil/Quaternion Multiplication
  Quaternion Normalize : sharedutil/Quaternion Normalize  aMode=aMode
  Out1 : Outport
  wires:
  Quaternion Multiplication/1 -> (q0,q1,q2,q3) to (q1,q2,q3,q0),/1(In1)
  "(q1,q2,q3,q0) to (q0,q1,q2,q3) "/1(Out1) -> Quaternion Normalize/1
  Q_input1/1 -> (q1,q2,q3,q0) to (q0,q1,q2,q3) 1/1(Q_input)
  (q1,q2,q3,q0) to (q0,q1,q2,q3) 1/1(Out1) -> Quaternion Multiplication/2
  (q0,q1,q2,q3) to (q1,q2,q3,q0),/1(Out1) -> Out1/1
  Q_input/1 -> "(q1,q2,q3,q0) to (q0,q1,q2,q3) "/1(Q_input)
  Quaternion Normalize/1 -> Quaternion Multiplication/1

== system SimulatorSpencer/Mode Logic /Slew Mode/ACS/w (q1,q2,q3,q0) to (q0,q1,q2,q3)  ==
  y : Inport
  Vector Concatenate : Concatenate
  e_q_vect1 : Selector  InputPortWidth=4  IndexOptions=Index vector (dialog)  Indices=[1 2 3]  OutputSizes=1
  e_q_vect2 : Selector  InputPortWidth=4  IndexOptions=Index vector (dialog)  Indices=[4]  OutputSizes=1
  Out1 : Outport
  wires:
  Vector Concatenate/1 -> Out1/1
  e_q_vect1/1 -> Vector Concatenate/2
  e_q_vect2/1 -> Vector Concatenate/1
  y/1 -> e_q_vect1/1, e_q_vect2/1

== system SimulatorSpencer/Mode Logic /Slew Mode/DCM to Axis-Angle/a1 ==
  In1 : Inport
  Input : Inport  Port=2
  phi : Inport  Port=3
  Display : Display
  Divide : Product  Inputs=*/
  Minus : Sum  Inputs=+-
  Multiply : Gain  Gain=2
  Sin : Trigonometry
  a1 : Outport
  wires:
  In1/1 -> Minus/1
  Input/1 -> Minus/2
  phi/1 -> Sin/1
  Sin/1 -> Multiply/1
  Divide/1 -> a1/1
  Multiply/1 -> Divide/2
  Minus/1 -> Display/1, Divide/1

== system SimulatorSpencer/Mode Logic /Slew Mode/DCM to Axis-Angle/a2 ==
  In1 : Inport
  Input : Inport  Port=2
  phi : Inport  Port=3
  Display : Display
  Divide : Product  Inputs=*/
  Minus : Sum  Inputs=+-
  Multiply : Gain  Gain=2
  Sin : Trigonometry
  a2 : Outport
  wires:
  In1/1 -> Minus/1
  Input/1 -> Minus/2
  phi/1 -> Sin/1
  Sin/1 -> Multiply/1
  Divide/1 -> a2/1
  Multiply/1 -> Divide/2
  Minus/1 -> Display/1, Divide/1

== system SimulatorSpencer/Mode Logic /Slew Mode/DCM to Axis-Angle/a3 ==
  In1 : Inport
  Input : Inport  Port=2
  phi : Inport  Port=3
  Display : Display
  Divide : Product  Inputs=*/
  Minus : Sum  Inputs=+-
  Multiply : Gain  Gain=2
  Sin : Trigonometry
  a3 : Outport
  wires:
  In1/1 -> Minus/1
  Input/1 -> Minus/2
  phi/1 -> Sin/1
  Sin/1 -> Multiply/1
  Divide/1 -> a3/1
  Multiply/1 -> Divide/2
  Minus/1 -> Display/1, Divide/1

== system SimulatorSpencer/Mode Logic /Slew Mode/DCM to Axis-Angle/phi ==
  In1 : Inport
  Input : Inport  Port=2
  Input1 : Inport  Port=3
  Acos : Trigonometry  Operator=acos
  Add : Sum  Inputs=++++
  Constant : Constant  Value=-1
  Multiply : Gain  Gain=0.5
  phi : Outport
  wires:
  Input1/1 -> Add/3
  Input/1 -> Add/2
  In1/1 -> Add/1
  Constant/1 -> Add/4
  Add/1 -> Multiply/1
  Multiply/1 -> Acos/1
  Acos/1 -> phi/1

== system SimulatorSpencer/Mode Logic /Slew Mode/DCM to Axis-Angle3/(q1,q2,q3,q0) to (q0,q1,q2,q3)  ==
  Q_input : Inport
  Vector Concatenate : Concatenate
  e_q_vect1 : Selector  InputPortWidth=4  IndexOptions=Index vector (dialog)  Indices=[1 2 3]  OutputSizes=1
  e_q_vect2 : Selector  InputPortWidth=4  IndexOptions=Index vector (dialog)  Indices=[4]  OutputSizes=1
  Out1 : Outport
  wires:
  Q_input/1 -> e_q_vect2/1, e_q_vect1/1
  e_q_vect2/1 -> Vector Concatenate/1
  e_q_vect1/1 -> Vector Concatenate/2
  Vector Concatenate/1 -> Out1/1

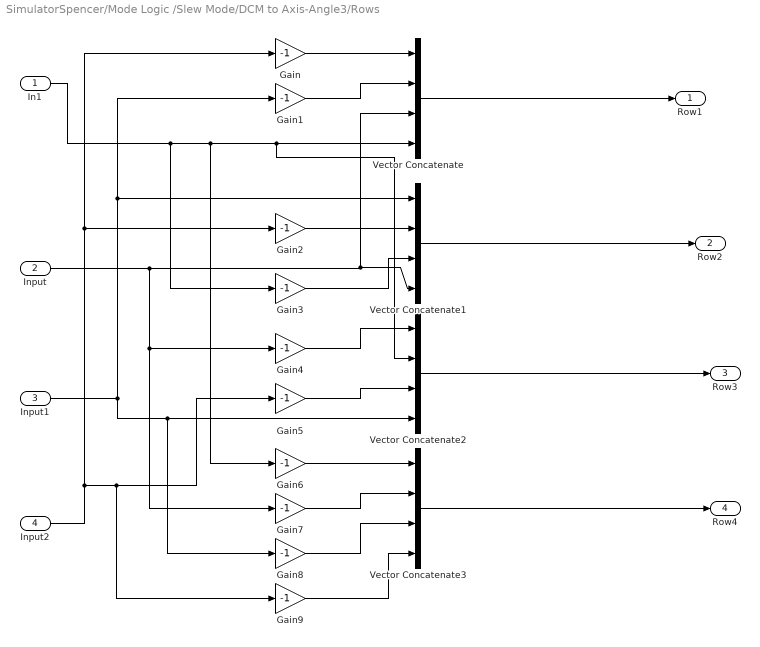
== system SimulatorSpencer/Mode Logic /Slew Mode/DCM to Axis-Angle3/Rows ==
  In1 : Inport
  Input : Inport  Port=2
  Input1 : Inport  Port=3
  Input2 : Inport  Port=4
  Gain{,1..9} (10 alike) : Gain  Gain=-1
  Vector Concatenate{,1..3} (4 alike) : Concatenate  NumInputs=4
  Row1 : Outport
  Row2 : Outport  Port=2
  Row3 : Outport  Port=3
  Row4 : Outport  Port=4
  wires:
  Vector Concatenate/1 -> Row1/1
  Vector Concatenate1/1 -> Row2/1
  Vector Concatenate2/1 -> Row3/1
  Vector Concatenate3/1 -> Row4/1
  Input2/1 -> Gain9/1, Gain5/1, Gain2/1, Gain/1
  Gain/1 -> Vector Concatenate/1
  Input1/1 -> Vector Concatenate1/1, Gain1/1, Gain8/1, Vector Concatenate2/4
  Gain1/1 -> Vector Concatenate/2
  In1/1 -> Gain3/1, Gain6/1, Vector Concatenate2/2, Vector Concatenate/4
  Input/1 -> Gain7/1, Gain4/1, Vector Concatenate1/4, Vector Concatenate/3
  Gain2/1 -> Vector Concatenate1/2
  Gain3/1 -> Vector Concatenate1/3
  Gain4/1 -> Vector Concatenate2/1
  Gain5/1 -> Vector Concatenate2/3
  Gain6/1 -> Vector Concatenate3/1
  Gain7/1 -> Vector Concatenate3/2
  Gain8/1 -> Vector Concatenate3/3
  Gain9/1 -> Vector Concatenate3/4

== system SimulatorSpencer/Mode Logic /Slew Mode/For Loop/Enabled Subsystem ==
  In1 : Inport
  Enable : EnablePort
  Out1 : Outport
  wires:
  In1/1 -> Out1/1

== system SimulatorSpencer/Mode Logic /Slew Mode/For Loop/Subsystem ==
  Input : Inport
  Quaternions to Direction Cosine Matrix2 : sharedtransform/Quaternions to  Direction Cosine Matrix  Commented=on  aMode=aMode
      settings: LibrarySourceBlock=|
      | aerolibtransform2/Quaternions to
      | Direction Cosine Matrix
  Subsystem3 : Subsystem  Commented=on
  "w (q1,q2,q3,q0) to (q0,q1,q2,q3) " : Subsystem
      settings: PortSchema="{\"entries\":[{\"content\":{\"sides\":[{\"content\":{\"connectorIds\":[\"Out1\"]},\"type\":\"ConnectorPlacement.EquallySpacedRectSide\",\"uuid\":\"97b477ad-5663-4010-b344-d27b8ec095be\"},{\"content\":{\"connectorIds\":[\"In1\"],\"side\":\"RIGHT\"},\"type\":\"ConnectorPlacement.EquallySpacedRectSide\",\"uuid\":\"41fe4029-0263-4427-bdfc-3c26258b8a65\"},{\"content\":{\"side\":\"TOP\"},\"type\":\"ConnectorPlacement.EquallySpacedRectSide\",\"uuid\":\"9fb3a03d-539a-4245-bd7d-8174d3d0797f\"}]},\"type\":\"ConnectorPlacement.EquallySpacedConnector\",\"uuid\":\"44222554-f3ae-4bc6-b92c-7571a5ce84f7\"}],\"packageUris\":[\"http://schema.mathworks.com/mf0/Connector/R2020b\"],\"version\":\"1.0\"}"
  Angle (phi) : Outport
  wires:
  Quaternions to Direction Cosine Matrix2/1 -> Subsystem3/1(In1)
  Input/1 -> "w (q1,q2,q3,q0) to (q0,q1,q2,q3) "/1(y)
  "w (q1,q2,q3,q0) to (q0,q1,q2,q3) "/1(Angle (phi)) -> Angle (phi)/1

== system SimulatorSpencer/Mode Logic /Slew Mode/Subsystem/Quaternion Integration ==
  w_Body : Inport
  Integrator1 : Integrator  InitialCondition=q_init
  q_normalize : Subsystem
  qderiv : Subsystem
  q_I_Body : Outport
  wires:
  qderiv/1(qd) -> Integrator1/1
  Integrator1/1 -> q_normalize/1(q_in)
  q_normalize/1(q_out) -> q_I_Body/1, qderiv/2(q)
  w_Body/1 -> qderiv/1(w)

== system SimulatorSpencer/Mode Logic /Slew Mode/Subsystem/S ==
  Input : Inport
  Divide : Product  Inputs=*/
  Pi1 : Constant  Value=pi  OutDataTypeStr=Inherit: Inherit via back propagation
  Subtract1 : Sum  Commented=on  Inputs=+-
  "Total time " : Constant  Value=10
  Out1 : Outport
  wires:
  Divide/1 -> Out1/1
  Pi1/1 -> Divide/1
  Input/1 -> Subtract1/2
  "Total time "/1 -> Divide/2

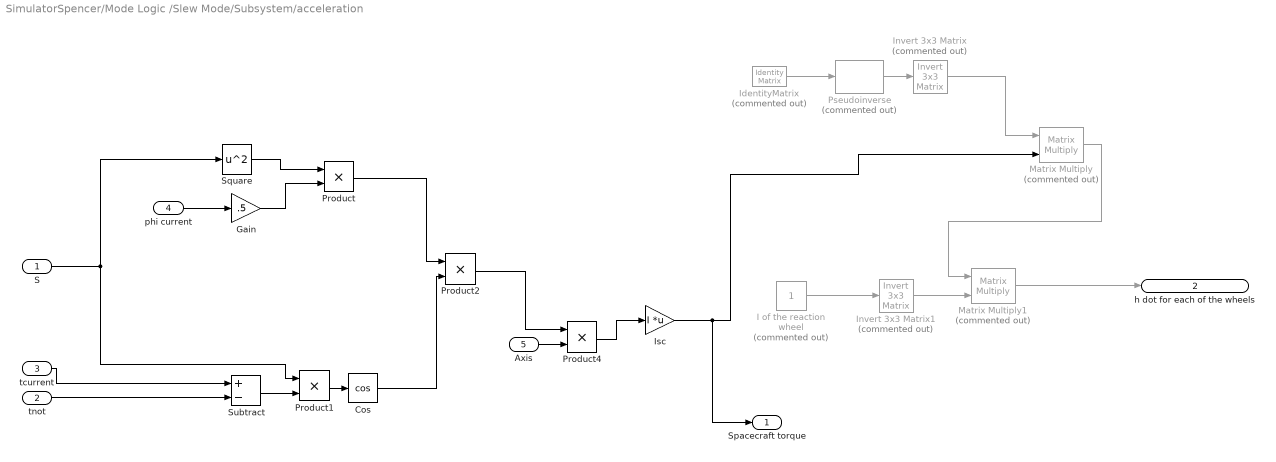
== system SimulatorSpencer/Mode Logic /Slew Mode/Subsystem/acceleration ==
  S : Inport
  tnot : Inport  Port=2
  tcurrent : Inport  Port=3
  phi current : Inport  Port=4
  Axis : Inport  Port=5
  Cos : Trigonometry  Operator=cos
  Gain : Gain  Gain=.5
  I of the reaction wheel : Constant  Commented=on
  IdentityMatrix : IdentityMatrix  Commented=on  OutputDimensions=3
  Invert 3x3 Matrix : aerolibutil/Invert  3x3 Matrix  Commented=on
  Invert 3x3 Matrix1 : aerolibutil/Invert  3x3 Matrix  Commented=on
  Isc : Gain  Gain=I  Multiplication=Matrix(K*u)
  Matrix Multiply : Product  Commented=on  Multiplication=Matrix(*)
  Matrix Multiply1 : Product  Commented=on  Multiplication=Matrix(*)
  Product{,1..2,4} (4 alike) : Product
  Pseudoinverse : dspinverses/Pseudoinverse  Commented=on  wanterr=off  SimulateUsing=Interpreted execution
  Square : Math  Operator=square
  Subtract : Sum  Inputs=+-
  Spacecraft torque : Outport
  h dot for each of the wheels : Outport  Port=2
  wires:
  S/1 -> Square/1, Product1/1
  Square/1 -> Product/1
  phi current/1 -> Gain/1
  Gain/1 -> Product/2
  tcurrent/1 -> Subtract/1
  tnot/1 -> Subtract/2
  Subtract/1 -> Product1/2
  Product1/1 -> Cos/1
  Product/1 -> Product2/1
  IdentityMatrix/1 -> Pseudoinverse/1
  Pseudoinverse/1 -> Invert 3x3 Matrix/1
  Invert 3x3 Matrix/1 -> Matrix Multiply/1
  Isc/1 -> Matrix Multiply/2, Spacecraft torque/1
  I of the reaction wheel/1 -> Invert 3x3 Matrix1/1
  Matrix Multiply/1 -> Matrix Multiply1/1
  Invert 3x3 Matrix1/1 -> Matrix Multiply1/2
  Cos/1 -> Product2/2
  Product2/1 -> Product4/1
  Axis/1 -> Product4/2
  Product4/1 -> Isc/1
  Matrix Multiply1/1 -> h dot for each of the wheels/1

== system SimulatorSpencer/Mode Logic /ACS/Free Rigid Body 1/Quaternion Integration/q_normalize ==
  q_in : Inport  PortDimensions=4
  Dot Product : DotProduct  OutDataTypeStr=Inherit: Inherit via internal rule
  Product : Product  Inputs=*/  InputSameDT=on  SaturateOnIntegerOverflow=on  OutDataTypeStr=Inherit: Same as first input
  SignedSqrt : Sqrt  IntermediateResultsDataTypeStr=double
  q_out : Outport
  wires:
  Product/1 -> q_out/1
  SignedSqrt/1 -> Product/2
  q_in/1 -> Dot Product/2, Dot Product/1, Product/1
  Dot Product/1 -> SignedSqrt/1

== system SimulatorSpencer/Mode Logic /ACS/Free Rigid Body 1/Quaternion Integration/qderiv ==
  w : Inport
  q : Inport  Port=2
  Mux : Mux  Inputs=2
  Mux1 : Mux
  qd1 : Fcn  Expr=(u(7)*u(1)-u(6)*u(2)+u(5)*u(3))/2
  qd2 : Fcn  Expr=(u(6)*u(1)+u(7)*u(2)-u(4)*u(3))/2
  qd3 : Fcn  Expr=(-u(5)*u(1)+u(4)*u(2)+u(7)*u(3))/2
  qd4 : Fcn  Expr=(-u(4)*u(1)-u(5)*u(2)-u(6)*u(3))/2
  qd : Outport
  wires:
  Mux1/1 -> qd/1
  qd4/1 -> Mux1/4
  qd3/1 -> Mux1/3
  qd2/1 -> Mux1/2
  qd1/1 -> Mux1/1
  Mux/1 -> qd4/1, qd3/1, qd2/1, qd1/1
  q/1 -> Mux/2
  w/1 -> Mux/1
